simulink model "simulink_model"  (R2020b)
settings: Solver=FixedStepAuto  StartTime=0.0  StopTime=75  FixedStep=0.0001  RelTol=1e-3
undefined symbols (not defined in the file): Tn, Ts
settings Model: Creator=kpiotr  LastModifiedBy=karid

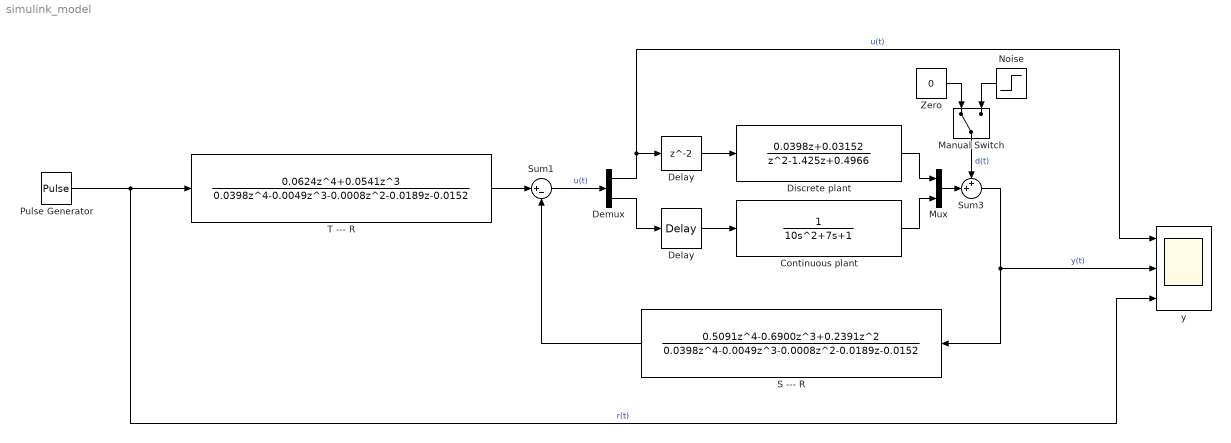
== system simulink_model ==
  Continuous plant : TransferFcn  Denominator=[10 7 1]
  Delay : TransportDelay  DelayTime=2  BufferSize=128000
  "Delay " : Delay  SampleTime=Ts
  Demux : Demux  Outputs=2
  Discrete plant : DiscreteTransferFcn  Numerator=[0.0398 0.03152]  Denominator=[1 -1.425 0.4966]  SampleTime=Ts
  Manual Switch : ManualSwitch
  Mux : Mux  Inputs=2
  Noise : Step  Time=30  SampleTime=0
  Pulse Generator : DiscretePulseGenerator  PulseType=Time based  Period=20 * Tn  PulseWidth=50  PhaseDelay=1
  S --- R : DiscreteTransferFcn  Numerator=[0.5091 -0.6900 0.2391 0 0]  Denominator=[0.0398 -0.0049 -0.0008 -0.0189 -0.0152]  SampleTime=Ts
  Sum1 : Sum  Inputs=|+-
  Sum3 : Sum  Inputs=++|
  T --- R : DiscreteTransferFcn  Description=""  Numerator=[0.0624 0.0541 0 0 0]  Denominator=[0.0398 -0.0049 -0.0008 -0.0189 -0.0152]  SampleTime=Ts
  Zero : Constant  Value=0  OutDataTypeStr=Inherit: Inherit via back propagation
  y : Scope  NumInputPorts=3
  wires:
  Pulse Generator/1 -> y/3, T --- R/1  "r(t)"
  Sum1/1 -> Demux/1  "u(t)"
  Sum3/1 -> S --- R/1, y/2  "y(t)"
  Delay/1 -> Continuous plant/1
  Discrete plant/1 -> Mux/1
  Demux/1 -> "Delay "/1, y/1  "u(t)"
  "Delay "/1 -> Discrete plant/1
  Continuous plant/1 -> Mux/2
  Mux/1 -> Sum3/2
  Demux/2 -> Delay/1
  S --- R/1 -> Sum1/2
  T --- R/1 -> Sum1/1
  Manual Switch/1 -> Sum3/1  "d(t)"
  Noise/1 -> Manual Switch/2
  Zero/1 -> Manual Switch/1
